simulink model "Zero"  (R2020b)
settings: Solver=VariableStepAuto  StartTime=0.0  StopTime=10.0  RelTol=1e-3
libraries: cstblocks x6
settings Model: Creator=Mah  LastModifiedBy=Mah

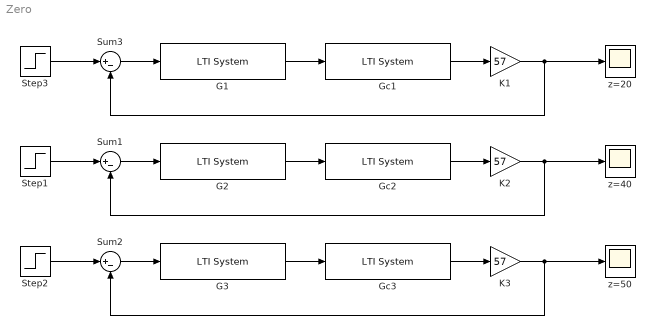
== system Zero ==
  G1 : cstblocks/LTI System  sys=tf(64.11 , [1 36.42 0])  IC=[]
  G2 : cstblocks/LTI System  sys=tf(64.11 , [1 36.42 0])  IC=[]
  G3 : cstblocks/LTI System  sys=tf(64.11 , [1 36.42 0])  IC=[]
  Gc1 : cstblocks/LTI System  sys=tf([1 20] , [1 87.6383])  IC=[]
  Gc2 : cstblocks/LTI System  sys=tf([1 40] , [1 87.6383])  IC=[]
  Gc3 : cstblocks/LTI System  sys=tf([1 50] , [1 87.6383])  IC=[]
  K1 : Gain  Gain=57
  K2 : Gain  Gain=57
  K3 : Gain  Gain=57
  Step1 : Step  Time=0  SampleTime=0
  Step2 : Step  Time=0  SampleTime=0
  Step3 : Step  Time=0  SampleTime=0
  Sum1 : Sum  Inputs=|+-
  Sum2 : Sum  Inputs=|+-
  Sum3 : Sum  Inputs=|+-
  z=20 : Scope
  z=40 : Scope
  z=50 : Scope
  wires:
  K2/1 -> z=40/1, Sum1/2
  Gc2/1 -> K2/1
  G2/1 -> Gc2/1
  Sum1/1 -> G2/1
  Step1/1 -> Sum1/1
  K3/1 -> z=50/1, Sum2/2
  Gc3/1 -> K3/1
  G3/1 -> Gc3/1
  Sum2/1 -> G3/1
  Step2/1 -> Sum2/1
  K1/1 -> z=20/1, Sum3/2
  Gc1/1 -> K1/1
  G1/1 -> Gc1/1
  Sum3/1 -> G1/1
  Step3/1 -> Sum3/1
